simulink library "Electrical_Library"  (R2014b)
settings: Solver=ode15s  StartTime=0.0  StopTime=10.0  RelTol=1e-3
libraries: fl_lib x7, elec_lib x3, nesl_utility x2, simulink x1
settings Model: Creator=ssekkai  LastModifiedBy=dmartins

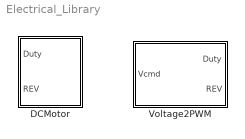
== system Electrical_Library ==
  " DCMotor" : Subsystem
      mask Display: image(imread('motor.jpg'))
  Voltage2PWM : Subsystem

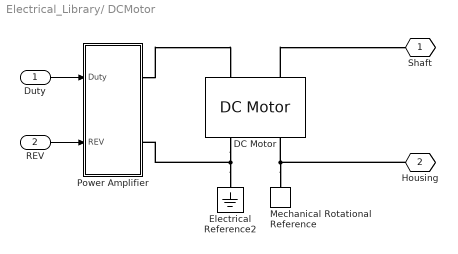
== system Electrical_Library/ DCMotor ==
  Duty : Inport
  REV : Inport  Port=2
  DC Motor : elec_lib/Actuators & Drivers/Rotational Actuators/DC Motor  parameterization=3  Ra=3.9 Ohm  La=0.001 H  emf_or_torque=1  Kv=1/7000 V/rpm  Ki=6.876e-04 N*m/A  T_stall=2.4e-04 N*m  w_max=4*7000 rpm  w_rated=25000 rpm  P_rated=10 W  V_rated=4 V  J=2 g*cm^2  lam_param=1  lam=1e-06 N*m/(rad/s)  i_noload=0 A  V_i_noload=1.5 V  speed0=0 rpm  alpha=0.00393 1/K  Tmeas=25 C  thermal_mass=100 J/K  initial_temperature=25 C
  Electrical Reference2 : fl_lib/Electrical/Electrical Elements/Electrical Reference
  Mechanical Rotational Reference : fl_lib/Mechanical/Rotational Elements/Mechanical Rotational Reference
  Power Amplifier : Subsystem
  Shaft : PMIOPort  Tag=PMCPort  Port=1  Side=Right
  Housing : PMIOPort  Tag=PMCPort  Port=2  Side=Right
  wires:
  Duty/1 -> Power Amplifier/1(Duty)
  REV/1 -> Power Amplifier/2(REV)
  connections:
  Power Amplifier/RConn1 -- DC Motor/LConn1
  DC Motor/LConn2 -- Shaft/RConn1
  Electrical Reference2/LConn1 -- DC Motor/RConn1 -- Power Amplifier/RConn2
  Mechanical Rotational Reference/LConn1 -- Housing/RConn1 -- DC Motor/RConn2

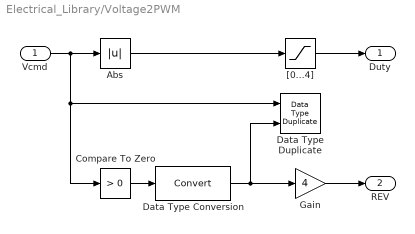
== system Electrical_Library/Voltage2PWM ==
  Vcmd : Inport
  Abs : Abs
  Compare To Zero : simulink/Logic and Bit Operations/Compare To Zero  relop=>  OutDataTypeStr=uint8
  Data Type Duplicate : DataTypeDuplicate
  Data Type Conversion : DataTypeConversion
  Gain : Gain  Gain=4
  "[0...4]" : Saturate  UpperLimit=4  LowerLimit=0
  Duty : Outport
  REV : Outport  Port=2
  wires:
  Abs/1 -> "[0...4]"/1
  Vcmd/1 -> Compare To Zero/1, Data Type Duplicate/1, Abs/1
  "[0...4]"/1 -> Duty/1
  Gain/1 -> REV/1
  Compare To Zero/1 -> Data Type Conversion/1
  Data Type Conversion/1 -> Data Type Duplicate/2, Gain/1

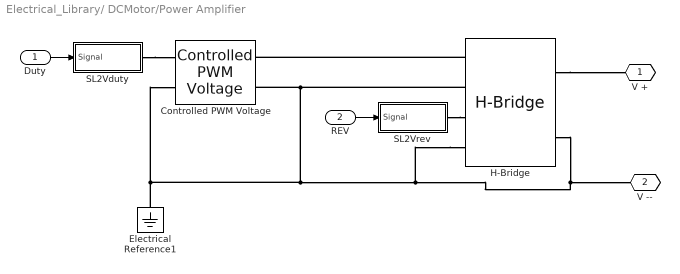
== system Electrical_Library/ DCMotor/Power Amplifier ==
  Duty : Inport
  REV : Inport  Port=2
  Controlled PWM Voltage : elec_lib/Actuators & Drivers/Drivers/Controlled PWM Voltage  F=4000 Hz  TD=0 s  pulse_width_offset=0 s  Vmin=0 V  Vmax=4 V  Vm=5 V  pwm_or_av=2  event_type=1  sample_time=1e-6 s
  Electrical Reference1 : fl_lib/Electrical/Electrical Elements/Electrical Reference
  H-Bridge : elec_lib/Actuators & Drivers/Drivers/H-Bridge  Venable=2.5 V  Vmax=5 V  Vreverse=2.5 V  Vbrake=2.5 V  Vm=4 V  pwm_or_av=2  discontinuous=0  freewheeling_mode=1  freewheeling_mode_disc=1  Ron=0.1 Ohm  Don=0.1 Ohm  Rload=10 Ohm  Lload=1e-5 H  F=10 kHz  w_vec=[1, 2] s  i_vec=[1, 2] A  vMatrix=[1, 2; 3, 4] V
  SL2Vduty : Subsystem
  SL2Vrev : Subsystem
  V + : PMIOPort  Tag=PMCPort  Port=1  Side=Right
  V -- : PMIOPort  Tag=PMCPort  Port=2  Side=Right
  wires:
  Duty/1 -> SL2Vduty/1(Signal)
  REV/1 -> SL2Vrev/1(Signal)
  connections:
  H-Bridge/LConn4 -- V --/RConn1 -- H-Bridge/RConn2 -- H-Bridge/LConn2 -- Controlled PWM Voltage/RConn2 -- Electrical Reference1/LConn1 -- Controlled PWM Voltage/LConn2
  SL2Vrev/RConn1 -- H-Bridge/LConn3
  H-Bridge/RConn1 -- V +/RConn1
  SL2Vduty/RConn1 -- Controlled PWM Voltage/LConn1
  H-Bridge/LConn1 -- Controlled PWM Voltage/RConn1

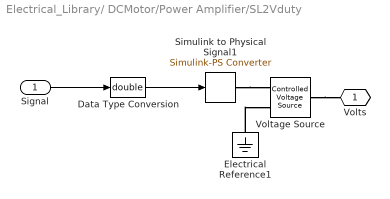
== system Electrical_Library/ DCMotor/Power Amplifier/SL2Vduty ==
  Signal : Inport
  Data Type Conversion : DataTypeConversion  OutDataTypeStr=double
  Electrical Reference1 : fl_lib/Electrical/Electrical Elements/Electrical Reference
  Simulink to Physical Signal1 : nesl_utility/Simulink-PS Converter  PhysicalDomain=network_engine_domain  SubClassName=ps_input  LeftPortType=input  RightPortType=output  PseudoPeriodic=off  Frequencies=[]  NoiseDistribution=none  NoiseParameters=[]  Unit=V  AffineConversion=off  InputFiltering=off  SimscapeFilterOrder=1  InputFilterTimeConstant=.001  UdotUserProvided=0
  Voltage Source : fl_lib/Electrical/Electrical Sources/Controlled Voltage Source
  Volts : PMIOPort  Tag=PMCPort  Port=1  Side=Right
  wires:
  Signal/1 -> Data Type Conversion/1
  Data Type Conversion/1 -> Simulink to Physical Signal1/1
  connections:
  Voltage Source/LConn1 -- Volts/RConn1
  Simulink to Physical Signal1/RConn1 -- Voltage Source/RConn1
  Electrical Reference1/LConn1 -- Voltage Source/RConn2

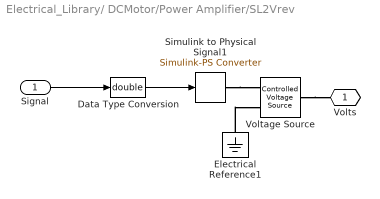
== system Electrical_Library/ DCMotor/Power Amplifier/SL2Vrev ==
  Signal : Inport
  Data Type Conversion : DataTypeConversion  OutDataTypeStr=double
  Electrical Reference1 : fl_lib/Electrical/Electrical Elements/Electrical Reference
  Simulink to Physical Signal1 : nesl_utility/Simulink-PS Converter  PhysicalDomain=network_engine_domain  SubClassName=ps_input  LeftPortType=input  RightPortType=output  PseudoPeriodic=off  Frequencies=[]  NoiseDistribution=none  NoiseParameters=[]  Unit=V  AffineConversion=off  InputFiltering=off  SimscapeFilterOrder=1  InputFilterTimeConstant=.001  UdotUserProvided=0
  Voltage Source : fl_lib/Electrical/Electrical Sources/Controlled Voltage Source
  Volts : PMIOPort  Tag=PMCPort  Port=1  Side=Right
  wires:
  Signal/1 -> Data Type Conversion/1
  Data Type Conversion/1 -> Simulink to Physical Signal1/1
  connections:
  Electrical Reference1/LConn1 -- Voltage Source/RConn2
  Simulink to Physical Signal1/RConn1 -- Voltage Source/RConn1
  Voltage Source/LConn1 -- Volts/RConn1
